simulink model "Harrier_noObserver"  (R2020a)
settings: Solver=VariableStepAuto  StartTime=0.0  StopTime=100  RelTol=1e-3
values from neighbouring files (symbols this model uses):
  A = [0, 0, 1, 0 ... (first row only)    [HarrierLateralController.m]    (also in HarrierVerticalController.m)
  B = [0 ... (first row only)    [HarrierLateralController.m]    (also in HarrierVerticalController.m)
  K = [0.8,1,1,1].*K    [HarrierLateralController.m]    (also in HarrierVerticalController.m = place(A,B,roots_scaled))
  m = 22471    [HarrierLateralController.m]    (also in HarrierVerticalController.m)
  r = 0    [HarrierLateralController.m]    (also in HarrierVerticalController.m = [5*WS, 0, 0, 0])
settings Model: Creator=oscar  LastModifiedBy=Finn
settings DebuggingCC: SFMachineParentedDataDiag=error

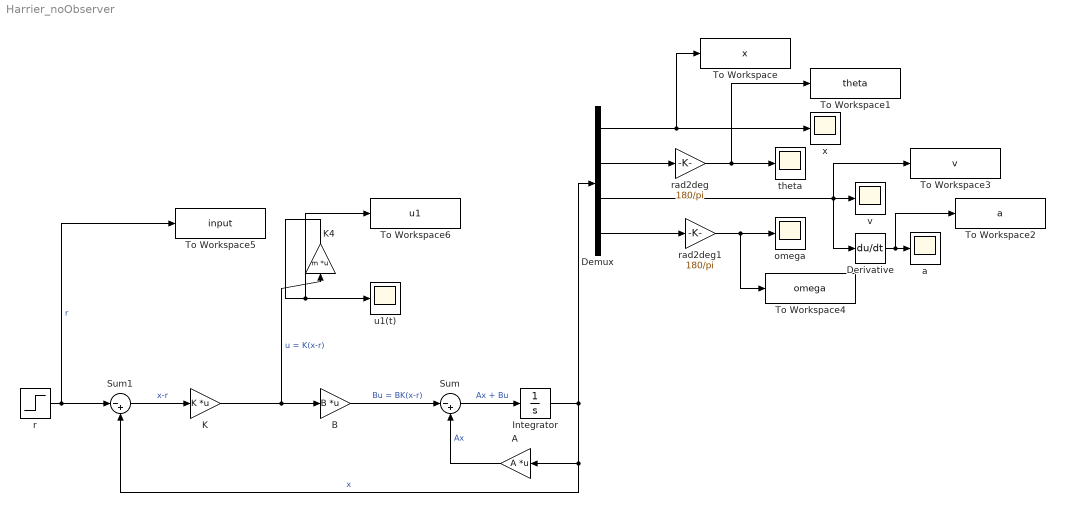
== system Harrier_noObserver ==
  A : Gain  Gain=A  Multiplication=Matrix(K*u)
  B : Gain  Gain=B  Multiplication=Matrix(K*u)
  Demux : Demux
  Derivative : Derivative
  Integrator : Integrator
  K : Gain  Gain=K  Multiplication=Matrix(K*u)
  K4 : Gain  Gain=m  Multiplication=Matrix(K*u)
  Sum : Sum  Inputs=|-+
  Sum1 : Sum  Inputs=|-+
  To Workspace : ToWorkspace  VariableName=x  SampleTime=-1
  To Workspace1 : ToWorkspace  VariableName=theta  SampleTime=-1
  To Workspace2 : ToWorkspace  VariableName=a  SampleTime=-1
  To Workspace3 : ToWorkspace  VariableName=v  SampleTime=-1
  To Workspace4 : ToWorkspace  VariableName=omega  SampleTime=-1
  To Workspace5 : ToWorkspace  VariableName=input  SampleTime=-1
  To Workspace6 : ToWorkspace  VariableName=u1  SampleTime=-1
  a : Scope
  omega : Scope
  r : Step  Time=0  After=r  SampleTime=0
  rad2deg : Gain  Gain=180/pi
  rad2deg1 : Gain  Gain=180/pi
  theta : Scope
  u1(t) : Scope
  v : Scope
  x : Scope
  wires:
  Sum1/1 -> K/1  "x-r"
  B/1 -> Sum/1  "Bu = BK(x-r)"
  Sum/1 -> Integrator/1  "Ax + Bu"
  Demux/1 -> x/1, To Workspace/1
  Demux/2 -> rad2deg/1
  Demux/3 -> To Workspace3/1, Derivative/1, v/1
  Demux/4 -> rad2deg1/1
  A/1 -> Sum/2  "Ax"
  rad2deg/1 -> To Workspace1/1, theta/1
  rad2deg1/1 -> To Workspace4/1, omega/1
  Derivative/1 -> To Workspace2/1, a/1
  r/1 -> Sum1/1, To Workspace5/1  "r"
  Integrator/1 -> Demux/1, Sum1/2, A/1  "x"
  K/1 -> B/1, K4/1  "u = K(x-r)"
  K4/1 -> To Workspace6/1, u1(t)/1
